simulink model "example_window_Uvalue"  (R2016b)
settings: Solver=ode45  StartTime=8*3600  StopTime=9*3600  MaxStep=600  RelTol=1e-3  EnableMultiTasking=on
libraries: carnot x4
settings Model: Creator=drhf  LastModifiedBy=drhf
settings DataIOCC: LimitDataPoints=on  SaveFormat=Array
settings OptimizationCC: DefaultParameterBehavior=Inlined  LifeSpan=inf
settings DebuggingCC: UnderspecifiedInitializationDetection=Classic  MergeDetectMultiDrivingBlocksExec=none  SolverPrmCheckMsg=warning  SFUnexpectedBacktrackingDiag=warning  SFNoUnconditionalDefaultTransitionDiag=warning  SFExecutionAtInitializationDiag=none
settings HardwareCC: ProdBitPerPointer=32  ProdBitPerSizeT=32  ProdBitPerPtrDiffT=32  ProdLargestAtomicFloat=None  ProdIntDivRoundTo=Undefined  ProdEndianess=Unspecified  ProdWordSize=32  ProdHWDeviceType=32-bit Generic
settings ModelReferenceCC: PropagateSignalLabelsOutOfModel=off
settings GRTTargetCC: TargetLangStandard=C89/C90 (ANSI)  GeneratePreprocessorConditionals=Disable all
settings ConfigComp: CovMetricSettings=dw  CovHtmlReporting=on  CovSaveCumulativeToWorkspaceVar=on  CovSaveSingleToWorkspaceVar=on  CovExternalEMLEnable=off

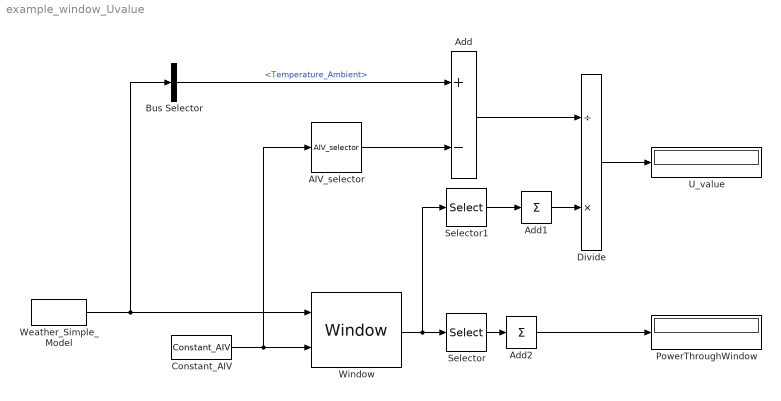
== system example_window_Uvalue ==
  AIV_selector : carnot/Outputs/AIV_selector  e1=on  e2=off  e3=off  e4=off  e5=off  e6=off  e7=off  e8=off  e9=off
  Add : Sum  Inputs=+-
  Add1 : Sum  Inputs=1
  Add2 : Sum  Inputs=1
  Bus Selector : BusSelector  OutputSignals=Temperature_Ambient
  Constant_AIV : carnot/Source/Ventilation/Constant_AIV  Tsens=20  Tcon=20  Trad=20  mw=0.012  mco=0.01  rhoair=1.2  cpair=1004  pair=100000  nair=0.5
  Divide : Product  Inputs=/*
  PowerThroughWindow : Display
  Selector : Selector  InputPortWidth=13  IndexOptions=Index vector (dialog)  Indices=[7 8]  OutputSizes=1
  Selector1 : Selector  InputPortWidth=13  IndexOptions=Index vector (dialog)  Indices=[7 8]  OutputSizes=1
  U_value : Display
  Weather_Simple_Model : carnot/Weather/Weather_Simple_Model  lat=60  Ibn=900  Idg=100  tamb=5  deltaTsky=-6  rh=50  precip="10e-3/24/3600           % 10 mm in 24 h"  cloud=0.125  p=1013e2  vw=1  wdir=270
  Window : carnot/Load/Houses/wall_floor/Window  windowsize=[1 1]  frame=0  pos=0  t0=20  d=[0.01 0.01]  cond=[0.4 0.4]  cwall=[0.28 0.28]*3600  rho=[2500 2500]  misc=[0.2 0.1 1 1]  gvalue=0.6  tau=100  dactive=[0.005 0.015]
  wires:
  Constant_AIV/1 -> Window/2, AIV_selector/1
  Window/1 -> Selector1/1, Selector/1
  Selector/1 -> Add2/1
  AIV_selector/1 -> Add/2
  Add/1 -> Divide/1
  Selector1/1 -> Add1/1
  Add1/1 -> Divide/2
  Divide/1 -> U_value/1
  Add2/1 -> PowerThroughWindow/1
  Weather_Simple_Model/1 -> Bus Selector/1, Window/1
  Bus Selector/1 -> Add/1  "<Temperature_Ambient>"
